simulink model "ueb1_A1_a_ver2"  (R2016a)
settings: Solver=VariableStepAuto  StartTime=0.0  StopTime=10.0  RelTol=1e-3
values from neighbouring files (symbols this model uses):
  c = 10    [ueb1.m]
  d = 0.5    [ueb1.m]
  m = 1    [ueb1.m]
settings Model: Creator=bachman0  LastModifiedBy=bachman0

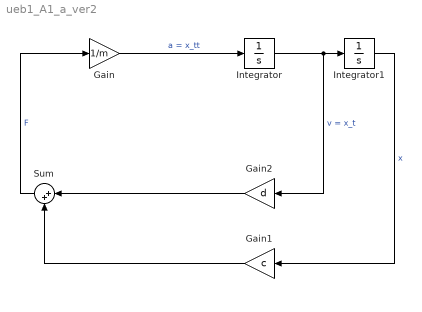
== system ueb1_A1_a_ver2 ==
  Gain : Gain  Gain=1/m
  Gain1 : Gain  Gain=c
  Gain2 : Gain  Gain=d
  Integrator : Integrator
  Integrator1 : Integrator
  Sum : Sum  Inputs=|++
  wires:
  Integrator/1 -> Gain2/1, Integrator1/1  "v = x_t"
  Gain/1 -> Integrator/1  "a = x_tt"
  Integrator1/1 -> Gain1/1  "x"
  Sum/1 -> Gain/1  "F"
  Gain2/1 -> Sum/1
  Gain1/1 -> Sum/2
